simulink model "Robot2dof_control_Friction_FullyTuned_RBFNN"  (Simulink 8.5)
settings: Solver=ode45  StartTime=0.0  StopTime=20  RelTol=1e-3
values from neighbouring files (symbols this model uses):
  l1 = 1    [Inv_Kinematic.m]    (also in Parameters.m)
  l2 = 0.5    [Inv_Kinematic.m]    (also in Parameters.m)
  m1 = 2    [Parameters.m]
  m2 = 1    [Parameters.m]
libraries: mblibv1 x13
(part 1 of 2)
settings Model: Creator=Le Tien Dung  LastModifiedBy=Administrator
settings DebuggingCC: FcnCallInpInsideContextMsg=UseLocalSettings
settings SimMechanicsCC: VisOnUpdateDiagram=on  VisDuringSimulation=on
settings ConfigurationSet: Description=SimMechanics 2G

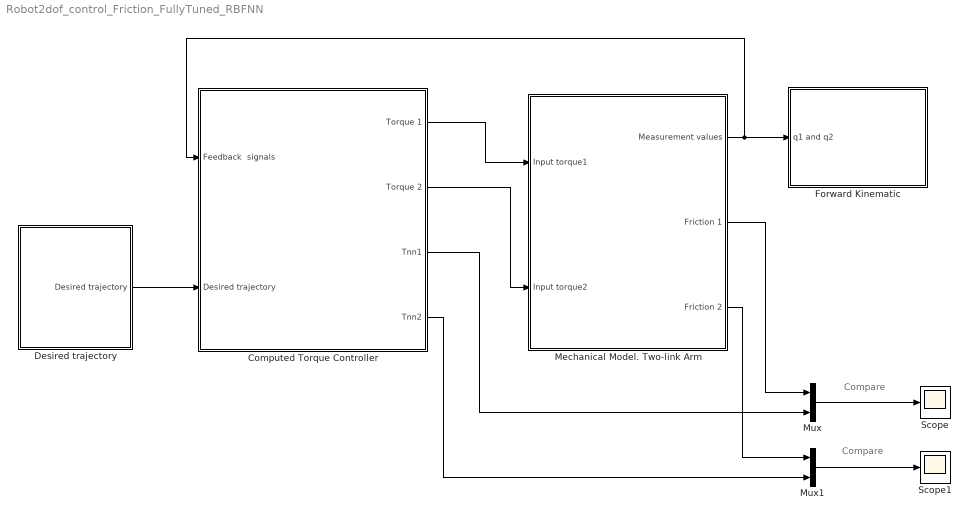
== system Robot2dof_control_Friction_FullyTuned_RBFNN ==
  note: Compare
  note: Compare
  Computed Torque Controller : Subsystem
  Desired trajectory : Subsystem
  Forward Kinematic : Subsystem
  Mechanical Model. Two-link Arm : Subsystem
  Mux : Mux  Inputs=2
  Mux1 : Mux  Inputs=2
  Scope : Scope
  Scope1 : Scope
      settings: SaveName=ScopeData2
  wires:
  Desired trajectory/1(Desired trajectory) -> Computed Torque Controller/2(Desired trajectory)
  Computed Torque Controller/1(Torque 1) -> Mechanical Model. Two-link Arm/1(Input torque1)
  Computed Torque Controller/2(Torque 2) -> Mechanical Model. Two-link Arm/2(Input torque2)
  Mux/1 -> Scope/1
  Mechanical Model. Two-link Arm/2(Friction 1) -> Mux/1
  Mux1/1 -> Scope1/1
  Mechanical Model. Two-link Arm/3(Friction 2) -> Mux1/1
  Mechanical Model. Two-link Arm/1(Measurement values) -> Computed Torque Controller/1(Feedback  signals), Forward Kinematic/1(q1 and q2)
  Computed Torque Controller/4(Tnn2) -> Mux1/2
  Computed Torque Controller/3(Tnn1) -> Mux/2

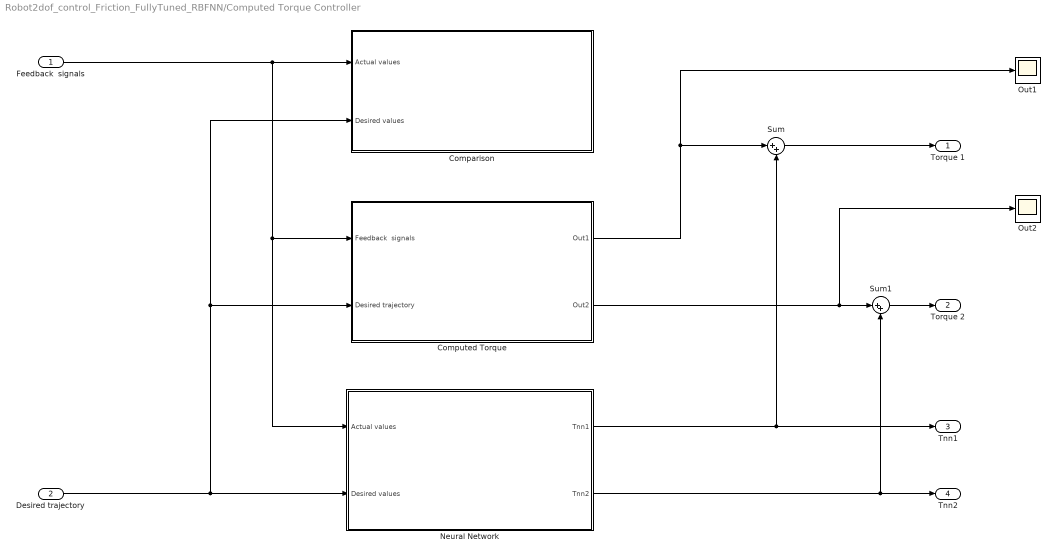
== system Robot2dof_control_Friction_FullyTuned_RBFNN/Computed Torque Controller ==
  Feedback  signals : Inport
  Desired trajectory : Inport  Port=2
  Comparison : Subsystem
  Computed Torque : Subsystem
  "Neural Network " : Subsystem
  Out1 : Scope
      settings: YMin=145.475  YMax=145.875  SaveName=Torque1
  Out2 : Scope
      settings: SaveName=Torque2
  Sum : Sum  Inputs=|++
  Sum1 : Sum  Inputs=|++
  Torque 1 : Outport
  Torque 2 : Outport  Port=2
  Tnn1 : Outport  Port=3
  Tnn2 : Outport  Port=4
  wires:
  Sum/1 -> Torque 1/1
  Sum1/1 -> Torque 2/1
  Computed Torque/1(Out1) -> Out1/1, Sum/1
  Computed Torque/2(Out2) -> Out2/1, Sum1/1
  Feedback  signals/1 -> Computed Torque/1(Feedback  signals), "Neural Network "/1("Actual values "), Comparison/1("Actual values ")
  Desired trajectory/1 -> "Neural Network "/2(Desired values), Comparison/2(Desired values), Computed Torque/2(Desired trajectory)
  "Neural Network "/1(Tnn1) -> Tnn1/1, Sum/2
  "Neural Network "/2(Tnn2) -> Tnn2/1, Sum1/2

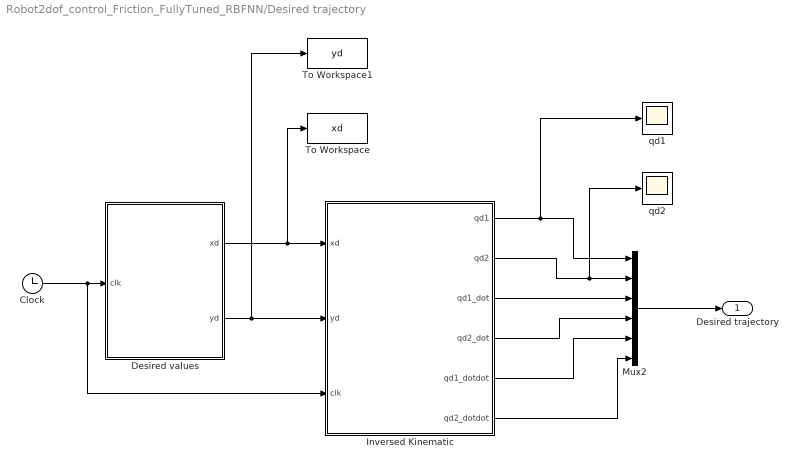
== system Robot2dof_control_Friction_FullyTuned_RBFNN/Desired trajectory ==
  " To Workspace1" : ToWorkspace  VariableName=yd  SaveFormat=Timeseries  SampleTime=-1
  Clock : Clock
  Desired values : MATLAB Function  TreatAsAtomicUnit=on
  Inversed Kinematic : MATLAB Function  TreatAsAtomicUnit=on
  Mux2 : Mux  Inputs=6
  To Workspace : ToWorkspace  VariableName=xd  SaveFormat=Timeseries  SampleTime=-1
  qd1 : Scope
  qd2 : Scope
      settings: SaveName=ScopeData3
  Desired trajectory : Outport
  wires:
  Mux2/1 -> Desired trajectory/1
  Desired values/1(xd) -> Inversed Kinematic/1(xd), To Workspace/1
  Clock/1 -> Desired values/1(clk), Inversed Kinematic/3(clk)
  Desired values/2(yd) -> Inversed Kinematic/2(yd), " To Workspace1"/1
  Inversed Kinematic/1(qd1) -> qd1/1, Mux2/1
  Inversed Kinematic/2(qd2) -> qd2/1, Mux2/2
  Inversed Kinematic/3(qd1_dot) -> Mux2/3
  Inversed Kinematic/4(qd2_dot) -> Mux2/4
  Inversed Kinematic/5(qd1_dotdot) -> Mux2/5
  Inversed Kinematic/6(qd2_dotdot) -> Mux2/6

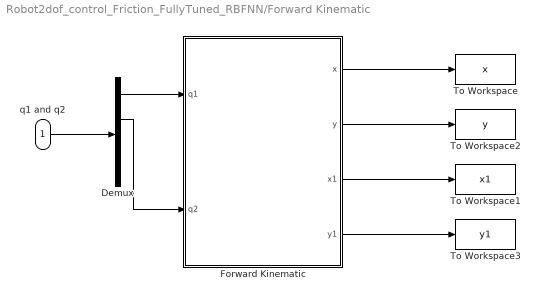
== system Robot2dof_control_Friction_FullyTuned_RBFNN/Forward Kinematic ==
  q1 and q2 : Inport
  Demux : Demux
  Forward Kinematic : MATLAB Function  TreatAsAtomicUnit=on
  To Workspace : ToWorkspace  VariableName=x  SaveFormat=Timeseries  SampleTime=-1
  To Workspace1 : ToWorkspace  VariableName=x1  SaveFormat=Timeseries  SampleTime=-1
  To Workspace2 : ToWorkspace  VariableName=y  SaveFormat=Timeseries  SampleTime=-1
  To Workspace3 : ToWorkspace  VariableName=y1  SaveFormat=Timeseries  SampleTime=-1
  wires:
  Forward Kinematic/4(y1) -> To Workspace3/1
  Demux/1 -> Forward Kinematic/1(q1)
  Forward Kinematic/2(y) -> To Workspace2/1
  Forward Kinematic/3(x1) -> To Workspace1/1
  Forward Kinematic/1(x) -> To Workspace/1
  Demux/2 -> Forward Kinematic/2(q2)
  q1 and q2/1 -> Demux/1

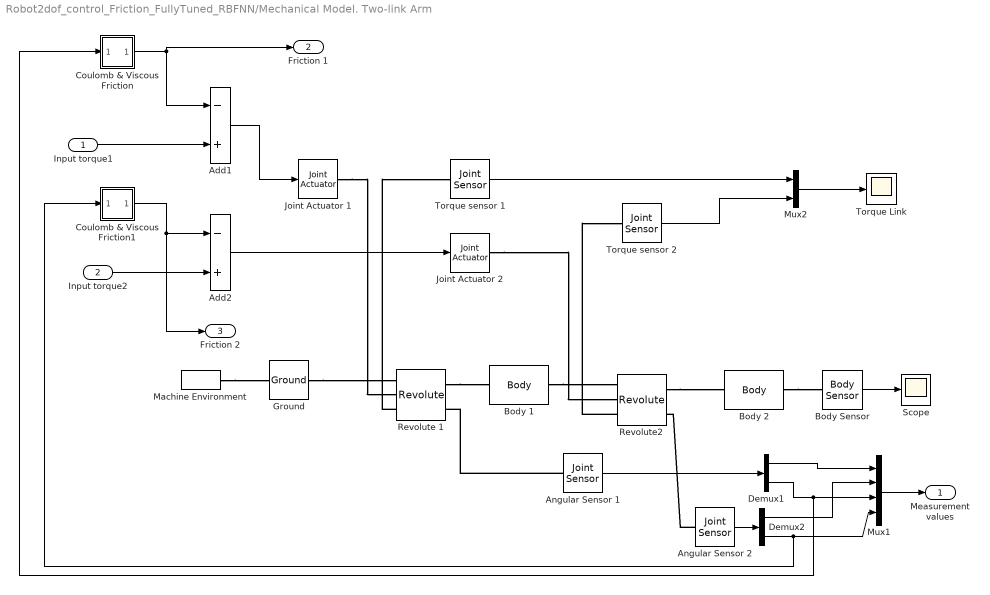
== system Robot2dof_control_Friction_FullyTuned_RBFNN/Mechanical Model. Two-link Arm ==
  Input torque1 : Inport
  Input torque2 : Inport  Port=2
  Add1 : Sum  Inputs=-+
  Add2 : Sum  Inputs=-+
  Angular Sensor 1 : mblibv1/Sensors &  Actuators/Joint Sensor  UpdateFromCAD=off  PhysicalDomain=Mechanical  PortType=blob  Muxed=on  Pose=off  Angle=on  AngleUnits=rad  ArcVelocity=on  ArcVelocityUnits=rad/s  ArcAcceleration=off  ArcAccelerationUnits=deg/s^2  CoordPosition=on  CoordPositionUnits=m  Velocity=off  VelocityUnits=m/s  Acceleration=off  AccelerationUnits=m/s^2  Quaternion=on  QuaternionDT=off  QuaternionDDT=off  QuaternionUnits=off  OutputVector=[1]  ActiveIO=on  Width=2  DialogClass=MechanicalSensorBlock  Primitive=R1  Force=off  ForceUnits=N  Torque=off  TorqueUnits=N*m  ReferenceFrame=Absolute (World)  ReactionSensedSide=Base  ReactionReferenceFrame=Absolute (World)  ReactionForce=off  ReactionForceUnits=N  ReactionMoment=off  ReactionMomentUnits=N*m
  Angular Sensor 2 : mblibv1/Sensors &  Actuators/Joint Sensor  UpdateFromCAD=off  PhysicalDomain=Mechanical  PortType=blob  Muxed=on  Pose=off  Angle=on  AngleUnits=rad  ArcVelocity=on  ArcVelocityUnits=rad/s  ArcAcceleration=off  ArcAccelerationUnits=deg/s^2  CoordPosition=on  CoordPositionUnits=m  Velocity=off  VelocityUnits=m/s  Acceleration=off  AccelerationUnits=m/s^2  Quaternion=on  QuaternionDT=off  QuaternionDDT=off  QuaternionUnits=off  OutputVector=[1]  ActiveIO=on  Width=2  DialogClass=MechanicalSensorBlock  Primitive=R1  Force=off  ForceUnits=N  Torque=off  TorqueUnits=N*m  ReferenceFrame=Absolute (World)  ReactionSensedSide=Base  ReactionReferenceFrame=Absolute (World)  ReactionForce=off  ReactionForceUnits=N  ReactionMoment=off  ReactionMomentUnits=N*m
  Body 1 : mblibv1/Bodies/Body  LConnTagsString=CS1  RConnTagsString=CS2  UpdateFromCAD=off  DialogClass=MechanicalBodyBlock  Mass=m1  MassUnits=kg  InertiaUnits=kg*m^2  Inertia=zeros(3,3)  Shape=Cylinder  ShapeDims=[1 1]  ShapeUnits=m  ShapeUse=false  Density=1  DensityUnits=kg/m^3  DensityUse=false  GraphicsMode=MACHINE_DEFAULT  BodyColorSelMode=MACHINE_DEFAULT  BodyColor=[1 0 0]  AttachedToCS=CG  CG=Left$CG$[l1/2 0 0]$World$World$m$[0 0 0]$Euler X-Y-Z$rad$World$false$none  WorkingFrames=Left$CS1$[0 0 0]$World$World$m$[0 0 0]$Euler X-Y-Z$rad$World$true$none#Right$CS2$[l1 0 0]$World$World$m$[0 0 0]$Euler X-Y-Z$rad$World$true$none  CGPos=[l1/2 0 0]  CGRot=[0 0 0]  CS0Pos=[]  CS0Rot=[]  CS1Pos=[0 0 0]  CS1Rot=[0 0 0]  CS2Pos=[l1 0 0]  CS2Rot=[0 0 0]  CS3Pos=[]  CS3Rot=[]  CS4Pos=[]  CS4Rot=[]  CS5Pos=[]  CS5Rot=[]  CS6Pos=[]  CS6Rot=[]  CS7Pos=[]  CS7Rot=[]  CS8Pos=[]  CS8Rot=[]  CS9Pos=[]  CS9Rot=[]  CS10Pos=[]  CS10Rot=[]  CS11Pos=[]  CS11Rot=[]  CS12Pos=[]  CS12Rot=[]  CS13Pos=[]  CS13Rot=[]  CS14Pos=[]  CS14Rot=[]  CS15Pos=[]  CS15Rot=[]  CS16Pos=[]  CS16Rot=[]  CS17Pos=[]  CS17Rot=[]  CS18Pos=[]  CS18Rot=[]  CS19Pos=[]  CS19Rot=[]  CS20Pos=[]  CS20Rot=[]
  Body 2 : mblibv1/Bodies/Body  LConnTagsString=CS1  RConnTagsString=CS2  UpdateFromCAD=off  DialogClass=MechanicalBodyBlock  Mass=m2  MassUnits=kg  InertiaUnits=kg*m^2  Inertia=zeros(3,3)  Shape=Cylinder  ShapeDims=[1 1]  ShapeUnits=m  ShapeUse=false  Density=1  DensityUnits=kg/m^3  DensityUse=false  GraphicsMode=MACHINE_DEFAULT  BodyColorSelMode=MACHINE_DEFAULT  BodyColor=[1 0 0]  AttachedToCS=CG  CG=Left$CG$[l2/2 0 0]$CS1$CS1$m$[0 0 0]$Euler X-Y-Z$rad$CS1$false$none  WorkingFrames=Left$CS1$[0 0 0]$Adjoining$Adjoining$m$[0 0 0]$Euler X-Y-Z$rad$Adjoining$true$none#Right$CS2$[l2 0 0]$CS1$CS1$m$[0 0 0]$Euler X-Y-Z$rad$CG$true$none  CGPos=[l2/2 0 0]  CGRot=[0 0 0]  CS0Pos=[]  CS0Rot=[]  CS1Pos=[0 0 0]  CS1Rot=[0 0 0]  CS2Pos=[l2 0 0]  CS2Rot=[0 0 0]  CS3Pos=[]  CS3Rot=[]  CS4Pos=[]  CS4Rot=[]  CS5Pos=[]  CS5Rot=[]  CS6Pos=[]  CS6Rot=[]  CS7Pos=[]  CS7Rot=[]  CS8Pos=[]  CS8Rot=[]  CS9Pos=[]  CS9Rot=[]  CS10Pos=[]  CS10Rot=[]  CS11Pos=[]  CS11Rot=[]  CS12Pos=[]  CS12Rot=[]  CS13Pos=[]  CS13Rot=[]  CS14Pos=[]  CS14Rot=[]  CS15Pos=[]  CS15Rot=[]  CS16Pos=[]  CS16Rot=[]  CS17Pos=[]  CS17Rot=[]  CS18Pos=[]  CS18Rot=[]  CS19Pos=[]  CS19Rot=[]  CS20Pos=[]  CS20Rot=[]
  Body Sensor : mblibv1/Sensors &  Actuators/Body Sensor  UpdateFromCAD=off  PhysicalDomain=Mechanical  PortType=blob  Muxed=on  Pose=off  Angle=on  AngleUnits=deg  ArcVelocity=off  ArcVelocityUnits=deg/s  ArcAcceleration=off  ArcAccelerationUnits=deg/s^2  CoordPosition=on  CoordPositionUnits=m  Velocity=off  VelocityUnits=m/s  Acceleration=off  AccelerationUnits=m/s^2  Quaternion=on  QuaternionDT=off  QuaternionDDT=off  QuaternionUnits=off  OutputVector=[1]  ActiveIO=on  Width=3  DialogClass=MechanicalSensorBlock  ReferenceFrame=Absolute (World)
  Coulomb & Viscous Friction : Subsystem  AncestorBlock=simulink/Discontinuities/Coulomb & Viscous Friction  mask(Coulombic and Viscous Friction){offset=0.3, gain=2}
      mask prompts: offset "Coulomb friction value (Offset):"; gain "Coefficient of viscous friction (Gain):"
      mask help:
      | A discontinuity offset at zero models coulomb friction.  Linear gain models viscous friction.
      | y = sign(x) * (Gain * abs(x) + Offset)
      mask init:
      | dblOffset = double(offset(1));
      | dblGain = double(gain(1));
      | x=max(dblOffset,dblGain+dblOffset);
      mask Help:
      | This block has a discontinuity
      | at zero and a linear gain afterward.
      | y= sign(x)*(Gain*abs(x)+Offset)
      mask Display:
      | plot([-1 0 0 1],[-dblGain-dblOffset, -dblOffset, ...
      |     dblOffset, dblGain+dblOffset],...
      |     [-1 1],[0 0],[0 0],[-x,x])
  Coulomb & Viscous Friction1 : Subsystem  AncestorBlock=simulink/Discontinuities/Coulomb & Viscous Friction  mask(Coulombic and Viscous Friction){offset=0.3, gain=2}
      mask prompts: offset "Coulomb friction value (Offset):"; gain "Coefficient of viscous friction (Gain):"
      mask help:
      | A discontinuity offset at zero models coulomb friction.  Linear gain models viscous friction.
      | y = sign(x) * (Gain * abs(x) + Offset)
      mask init:
      | dblOffset = double(offset(1));
      | dblGain = double(gain(1));
      | x=max(dblOffset,dblGain+dblOffset);
      mask Help:
      | This block has a discontinuity
      | at zero and a linear gain afterward.
      | y= sign(x)*(Gain*abs(x)+Offset)
      mask Display:
      | plot([-1 0 0 1],[-dblGain-dblOffset, -dblOffset, ...
      |     dblOffset, dblGain+dblOffset],...
      |     [-1 1],[0 0],[0 0],[-x,x])
  Demux1 : Demux  Outputs=2
  Demux2 : Demux  Outputs=2
  Ground : mblibv1/Bodies/Ground  UpdateFromCAD=off  LeftPortType=env  RightPortType=workingframe  PhysicalDomain=Mechanical  DialogClass=GroundBlock  CoordPosition=[0 0 0]  CoordPositionUnits=m  StateVectorMgrId=1  MachineId=[2 0]  ShowEnvPort=on  ParameterChecksum=[3725278248, 2799600244, 2519587858, 4125248297]  TopologyChecksum=[537926085, 4288578989, 2306256578, 2519465812]
  Joint Actuator 1 : mblibv1/Sensors &  Actuators/Joint Actuator  UpdateFromCAD=off  PhysicalDomain=Mechanical  PortType=blob  ActuationStyle=Force  AngleUnits=deg  ArcVelocityUnits=deg/s  ArcAccelerationUnits=deg/s^2  CoordPositionUnits=m  VelocityUnits=m/s  AccelerationUnits=m/s^2  ForceUnits=N  TorqueUnits=N*m  ActiveIO=on  Width=1  DialogClass=MechanicalActuatorBlock  Primitive=R1  ReferenceFrame=Absolute (World)
  Joint Actuator 2 : mblibv1/Sensors &  Actuators/Joint Actuator  UpdateFromCAD=off  PhysicalDomain=Mechanical  PortType=blob  ActuationStyle=Force  AngleUnits=deg  ArcVelocityUnits=deg/s  ArcAccelerationUnits=deg/s^2  CoordPositionUnits=m  VelocityUnits=m/s  AccelerationUnits=m/s^2  ForceUnits=N  TorqueUnits=N*m  ActiveIO=on  Width=1  DialogClass=MechanicalActuatorBlock  Primitive=R1  ReferenceFrame=Absolute (World)
  Machine Environment : mblibv1/Bodies/Machine Environment  PortType=env  PhysicalDomain=Mechanical  DialogTemplateClass=MECH.MachineEnvironment  SyncWhenCopied=off  Gravity=[0 -9.81 0]  GravityUnits=m/s^2  GravityAsSignal=off  Dimensionality=3D Only  AnalysisType=Forward dynamics  LinearAssemblyTolerance=1e-3  LinearAssemblyToleranceUnits=m  AngularAssemblyTolerance=1e-3  AngularAssemblyToleranceUnits=rad  ConstraintSolverType=Stabilizing  ConstraintRelTolerance=1e-4  ConstraintAbsTolerance=1e-4  UseRobustSingularityHandling=off  RedundancyAnalysisToleranceType=Automatically select tolerance  RedundancyAnalysisTolerance=1e-14  StatePerturbationType=Fixed  PerturbationSize=1e-5  VisualizeMachine=on  BodyVisualizationType=Use model default body geometries  BodyColorSelMode=Use model default  DefaultBodyColor=[1 0 0]
  Mux1 : Mux
  Mux2 : Mux  Inputs=2
  Revolute 1 : mblibv1/Joints/Revolute  LConnTagsString=__newl0|SA1|SA2  RConnTagsString=__newr0|SA1  UpdateFromCAD=off  NumSAPorts=3  CutJoint=off  MarkAsCut=off  Primitives=prismatic  PrimitiveProps=R1$World$[0 0 1]$revolute  DialogClass=JointBlock  R1Axis=[0 0 1]
  Revolute2 : mblibv1/Joints/Revolute  LConnTagsString=__newl0|SA1|SA2  RConnTagsString=__newr0|SA1  UpdateFromCAD=off  NumSAPorts=3  CutJoint=off  MarkAsCut=off  Primitives=prismatic  PrimitiveProps=R1$Base$[0 0 1]$revolute  DialogClass=JointBlock  R1Axis=[0 0 1]
  Scope : Scope
      settings: SaveName=ScopeData6
  Torque Link : Scope
      settings: SaveName=Torq1_task
  Torque sensor 1 : mblibv1/Sensors &  Actuators/Joint Sensor  UpdateFromCAD=off  PhysicalDomain=Mechanical  PortType=blob  Muxed=on  Pose=off  Angle=off  AngleUnits=rad  ArcVelocity=off  ArcVelocityUnits=rad/s  ArcAcceleration=off  ArcAccelerationUnits=deg/s^2  CoordPosition=on  CoordPositionUnits=m  Velocity=off  VelocityUnits=m/s  Acceleration=off  AccelerationUnits=m/s^2  Quaternion=on  QuaternionDT=off  QuaternionDDT=off  QuaternionUnits=off  OutputVector=[1]  ActiveIO=on  Width=1  DialogClass=MechanicalSensorBlock  Primitive=R1  Force=off  ForceUnits=N  Torque=on  TorqueUnits=N*m  ReferenceFrame=Absolute (World)  ReactionSensedSide=Base  ReactionReferenceFrame=Absolute (World)  ReactionForce=off  ReactionForceUnits=N  ReactionMoment=off  ReactionMomentUnits=N*m
  Torque sensor 2 : mblibv1/Sensors &  Actuators/Joint Sensor  UpdateFromCAD=off  PhysicalDomain=Mechanical  PortType=blob  Muxed=on  Pose=off  Angle=off  AngleUnits=rad  ArcVelocity=off  ArcVelocityUnits=rad/s  ArcAcceleration=off  ArcAccelerationUnits=deg/s^2  CoordPosition=on  CoordPositionUnits=m  Velocity=off  VelocityUnits=m/s  Acceleration=off  AccelerationUnits=m/s^2  Quaternion=on  QuaternionDT=off  QuaternionDDT=off  QuaternionUnits=off  OutputVector=[1]  ActiveIO=on  Width=1  DialogClass=MechanicalSensorBlock  Primitive=R1  Force=off  ForceUnits=N  Torque=on  TorqueUnits=N*m  ReferenceFrame=Absolute (World)  ReactionSensedSide=Base  ReactionReferenceFrame=Absolute (World)  ReactionForce=off  ReactionForceUnits=N  ReactionMoment=off  ReactionMomentUnits=N*m
  Measurement values : Outport
  Friction 1 : Outport  Port=2
  Friction 2 : Outport  Port=3
  wires:
  Angular Sensor 1/1 -> Demux1/1
  Angular Sensor 2/1 -> Demux2/1
  Mux2/1 -> Torque Link/1
  Torque sensor 2/1 -> Mux2/2
  Torque sensor 1/1 -> Mux2/1
  Demux1/1 -> Mux1/1
  Demux2/1 -> Mux1/2
  Demux1/2 -> Mux1/3, Coulomb & Viscous Friction/1(In1)
  Demux2/2 -> Mux1/4, Coulomb & Viscous Friction1/1(In1)
  Mux1/1 -> Measurement values/1
  Add1/1 -> Joint Actuator 1/1
  Coulomb & Viscous Friction/1(Out1) -> Add1/1, Friction 1/1
  Input torque1/1 -> Add1/2
  Input torque2/1 -> Add2/2
  Add2/1 -> Joint Actuator 2/1
  Coulomb & Viscous Friction1/1(Out1) -> Add2/1, Friction 2/1
  Body Sensor/1 -> Scope/1
  connections:
  Revolute 1/RConn1 -- Body 1/LConn1
  Body 1/RConn1 -- Revolute2/LConn1
  Machine Environment/RConn1 -- Ground/LConn1
  Ground/RConn1 -- Revolute 1/LConn1
  Joint Actuator 1/RConn1 -- Revolute 1/LConn2
  Joint Actuator 2/RConn1 -- Revolute2/LConn2
  Angular Sensor 1/LConn1 -- Revolute 1/RConn2
  Angular Sensor 2/LConn1 -- Revolute2/RConn2
  Revolute2/LConn3 -- Torque sensor 2/LConn1
  Revolute 1/LConn3 -- Torque sensor 1/LConn1
  Body 2/RConn1 -- Body Sensor/LConn1
  Revolute2/RConn1 -- Body 2/LConn1

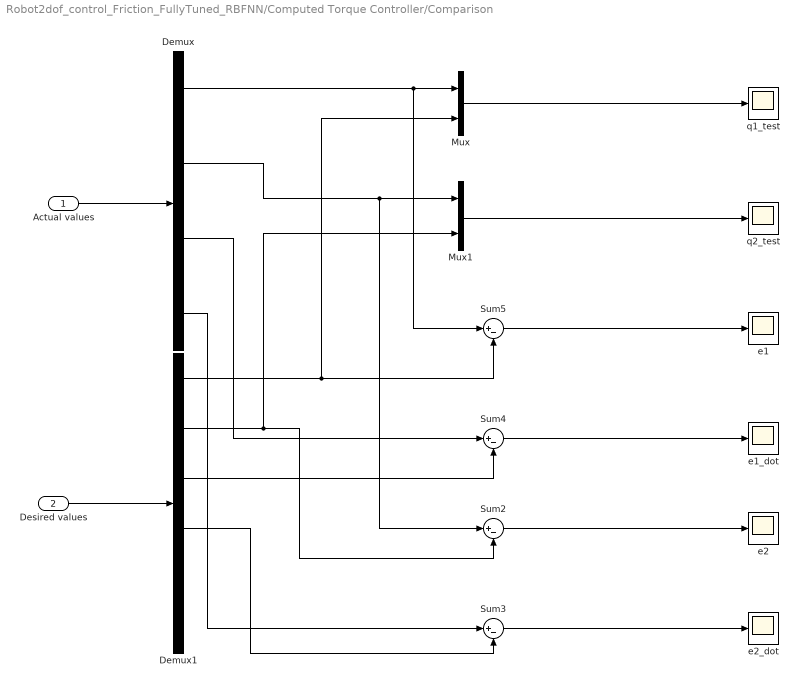
== system Robot2dof_control_Friction_FullyTuned_RBFNN/Computed Torque Controller/Comparison ==
  "Actual values " : Inport
  Desired values : Inport  Port=2
  Demux : Demux
  Demux1 : Demux  Outputs=6
  Mux : Mux  Inputs=2
  Mux1 : Mux  Inputs=2
  Sum{2..5} (4 alike) : Sum  Inputs=|+-
  e1 : Scope
      settings: ShowLegends=on  TimeRange=20  YMin=-1.4  YMax=0.3999999999999999  SaveName=Joint3
  e1_dot : Scope
      settings: TimeRange=20  YMin=-1  YMax=3  SaveName=Joint
  e2 : Scope
      settings: ShowLegends=on  TimeRange=19.57401979042055  YMin=-1.5  YMax=2.5  SaveName=Joint4
  e2_dot : Scope
      settings: YMax=3  SaveName=Joint5
  q1_test : Scope
      settings: ShowLegends=on  TimeRange=20  YMin=-0.002137407065588336  YMax=2  SaveName=Joint6
  q2_test : Scope
      settings: ShowLegends=on  TimeRange=20  YMin=-3.25  YMax=1.5  SaveName=Joint7
  wires:
  Mux1/1 -> q2_test/1
  Sum3/1 -> e2_dot/1
  Sum5/1 -> e1/1
  Sum4/1 -> e1_dot/1
  Sum2/1 -> e2/1
  Desired values/1 -> Demux1/1
  "Actual values "/1 -> Demux/1
  Mux/1 -> q1_test/1
  Demux/1 -> Sum5/1, Mux/1
  Demux1/1 -> Sum5/2, Mux/2
  Demux/2 -> Sum2/1, Mux1/1
  Demux1/2 -> Sum2/2, Mux1/2
  Demux/3 -> Sum4/1
  Demux1/3 -> Sum4/2
  Demux/4 -> Sum3/1
  Demux1/4 -> Sum3/2

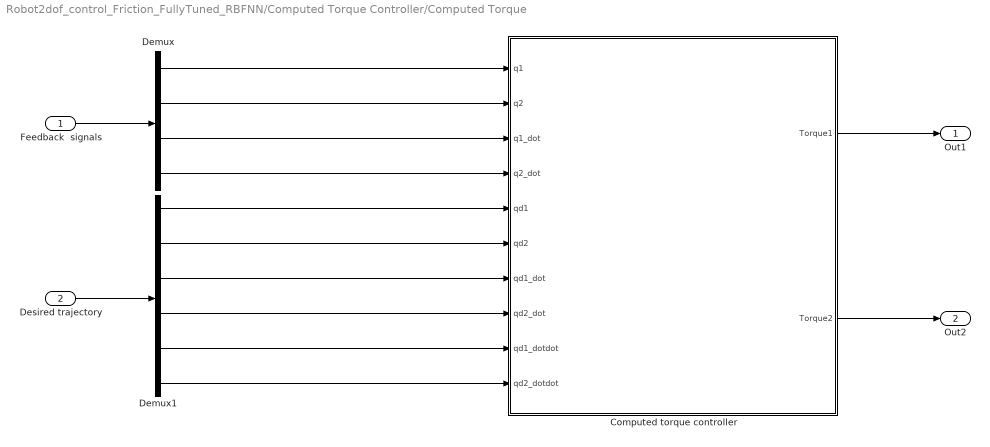
== system Robot2dof_control_Friction_FullyTuned_RBFNN/Computed Torque Controller/Computed Torque ==
  Feedback  signals : Inport
  Desired trajectory : Inport  Port=2
  Computed torque controller : MATLAB Function  TreatAsAtomicUnit=on
  Demux : Demux
  Demux1 : Demux  Outputs=6
  Out1 : Outport
  Out2 : Outport  Port=2
  wires:
  Computed torque controller/2(Torque2) -> Out2/1
  Computed torque controller/1(Torque1) -> Out1/1
  Demux/1 -> Computed torque controller/1(q1)
  Demux/2 -> Computed torque controller/2(q2)
  Demux/3 -> Computed torque controller/3(q1_dot)
  Demux/4 -> Computed torque controller/4(q2_dot)
  Demux1/1 -> Computed torque controller/5(qd1)
  Demux1/2 -> Computed torque controller/6(qd2)
  Demux1/3 -> Computed torque controller/7(qd1_dot)
  Demux1/4 -> Computed torque controller/8(qd2_dot)
  Demux1/5 -> Computed torque controller/9(qd1_dotdot)
  Demux1/6 -> Computed torque controller/10(qd2_dotdot)
  Feedback  signals/1 -> Demux/1
  Desired trajectory/1 -> Demux1/1

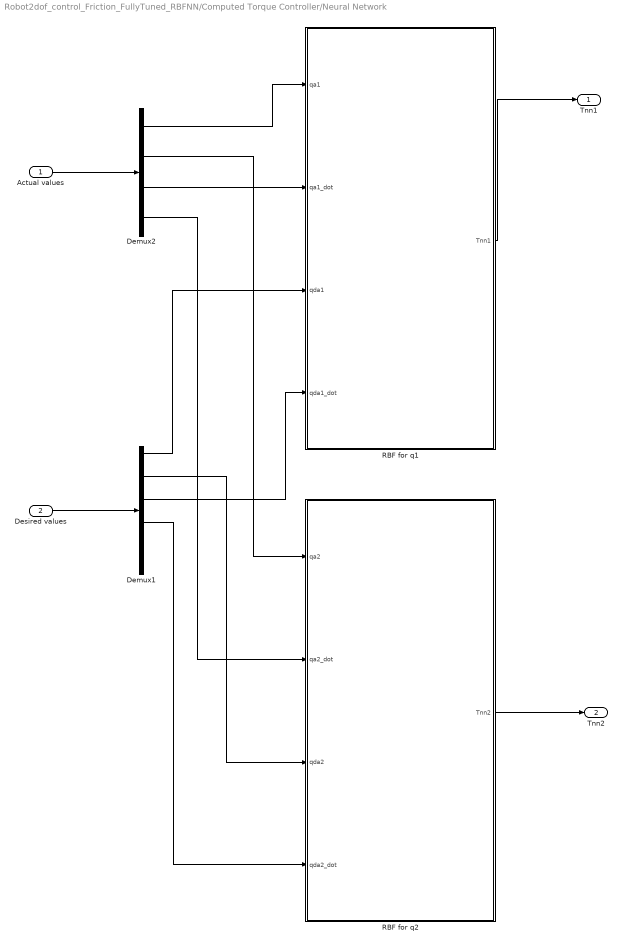
== system Robot2dof_control_Friction_FullyTuned_RBFNN/Computed Torque Controller/Neural Network  ==
  "Actual values " : Inport
  Desired values : Inport  Port=2
  Demux1 : Demux  Outputs=6
  Demux2 : Demux
  RBF for q1 : MATLAB Function  TreatAsAtomicUnit=on
  RBF for q2 : MATLAB Function  TreatAsAtomicUnit=on
  Tnn1 : Outport
  Tnn2 : Outport  Port=2
  wires:
  RBF for q1/1(Tnn1) -> Tnn1/1
  "Actual values "/1 -> Demux2/1
  RBF for q2/1(Tnn2) -> Tnn2/1
  Demux2/2 -> RBF for q2/1(qa2)
  Demux2/4 -> RBF for q2/2(qa2_dot)
  Demux2/1 -> RBF for q1/1(qa1)
  Demux2/3 -> RBF for q1/2(qa1_dot)
  Desired values/1 -> Demux1/1
  Demux1/1 -> RBF for q1/3(qda1)
  Demux1/4 -> RBF for q2/4(qda2_dot)
  Demux1/2 -> RBF for q2/3(qda2)
  Demux1/3 -> RBF for q1/4(qda1_dot)

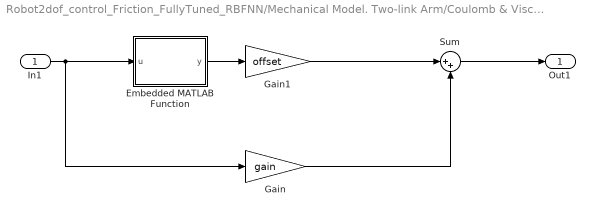
== system Robot2dof_control_Friction_FullyTuned_RBFNN/Mechanical Model. Two-link Arm/Coulomb & Viscous Friction ==
  In1 : Inport
  Embedded MATLAB Function : MATLAB Function  TreatAsAtomicUnit=on
  Gain : Gain  DisableCoverage=on  Gain=gain  SaturateOnIntegerOverflow=on  OutDataTypeStr=Inherit: Same as input
  Gain1 : Gain  DisableCoverage=on  Gain=offset  OutDataTypeStr=Inherit: Inherit via back propagation  SaturateOnIntegerOverflow=on
  Sum : Sum  Inputs=|++  SaturateOnIntegerOverflow=on  InputSameDT=on  OutDataTypeStr=Inherit: Same as first input
  Out1 : Outport
  wires:
  Embedded MATLAB Function/1(y) -> Gain1/1
  In1/1 -> Embedded MATLAB Function/1(u), Gain/1
  Gain1/1 -> Sum/1
  Sum/1 -> Out1/1
  Gain/1 -> Sum/2

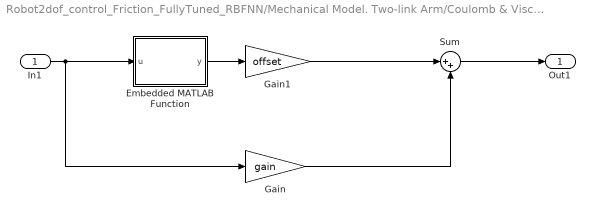
== system Robot2dof_control_Friction_FullyTuned_RBFNN/Mechanical Model. Two-link Arm/Coulomb & Viscous Friction1 ==
  In1 : Inport
  Embedded MATLAB Function : MATLAB Function  TreatAsAtomicUnit=on
  Gain : Gain  DisableCoverage=on  Gain=gain  SaturateOnIntegerOverflow=on  OutDataTypeStr=Inherit: Same as input
  Gain1 : Gain  DisableCoverage=on  Gain=offset  OutDataTypeStr=Inherit: Inherit via back propagation  SaturateOnIntegerOverflow=on
  Sum : Sum  Inputs=|++  SaturateOnIntegerOverflow=on  InputSameDT=on  OutDataTypeStr=Inherit: Same as first input
  Out1 : Outport
  wires:
  Gain/1 -> Sum/2
  Sum/1 -> Out1/1
  Gain1/1 -> Sum/1
  In1/1 -> Gain/1, Embedded MATLAB Function/1(u)
  Embedded MATLAB Function/1(y) -> Gain1/1

== matlab function Mechanical Model. Two-link Arm/Coulomb & Viscous Friction1/Embedded MATLAB Function ==
  data: u input double; y output double
function y = Sat(u)

if (abs(u)>0.01)
    y = sign(u);
else
    y = u/0.01;
end

== matlab function Desired trajectory/Desired values ==
  data: xd output double; yd output double; clk input double
function [xd, yd] = Desired_values(clk)
%% Parameters
T=5;
x0 = sqrt(2)/2;
y0 = sqrt(2)/2;
R = 0.5;
w = 2*pi/T;

%% Desired values
    xd = x0 + R*cos(w*clk +pi/2);
    yd = y0 + R*sin(w*clk +pi/2);
    
end

== matlab function Forward Kinematic/Forward Kinematic ==
  data: q1 input double; q2 input double; x output double; y output double; x1 output double; y1 output double
function [x,y,x1,y1]= Forward_Kinematic(q1, q2)
%% Parameters    
l1=1; 
l2=0.5;

%% Compute
x = l1*cos(q1) +l2*cos(q1+q2);
y = l1*sin(q1) +l2*sin(q1+q2);
x1 = l1*cos(q1);
y1 = l1*sin(q1);

== matlab function Desired trajectory/Inversed Kinematic ==
  data: xd input double; yd input double; qd1 output double; qd2 output double; qd1_dot output double; qd2_dot output double; clk input double; qd1_dotdot output double; qd2_dotdot output double
function [qd1, qd2, qd1_dot, qd2_dot, qd1_dotdot, qd2_dotdot] = InvKinematic( xd, yd, clk )
%% Parameters
x0 = sqrt(2)/2;
y0 = sqrt(2)/2;
l1 = 1;
l2 = 0.5;
T=5;
R = 0.5;
w = 2*pi/T;
x1 = 0;
y1= 0;
x = 0;
y= 0;
qd1 = 0;
qd2 = 0;


%% Inversed Kinematic
   qd2 = acos((xd^2 + yd^2 - l1^2 - l2^2)/(2*l1*l2));
   if(qd2 > 0)
       qd2 = -qd2;
       qd2_dot = ((2*pi*cos(pi/2 + (2*pi*clk)/5)*(sin(pi/2 + (2*pi*clk)/5)/2 + 2^(1/2)/2))/5 - (2*pi*sin(pi/2 + (2*pi*clk)/5)*(cos(pi/2 + (2*pi*clk)/5)/2 + 2^(1/2)/2))/5)/(- ((cos(pi/2 + (2*pi*clk)/5)/2 + 2^(1/2)/2)^2 + (sin(pi/2 + (2*pi*clk)/5)/2 + 2^(1/2)/2)^2 - 5/4)^2 + 1)^(1/2);
       qd2_dotdot = ((2*pi^2*sin(pi/2 + (2*pi*clk)/5)^2)/25 + (2*pi^2*cos(pi/2 + (2*pi*clk)/5)^2)/25 - (4*pi^2*cos(pi/2 + (2*pi*clk)/5)*(cos(pi/2 + (2*pi*clk)/5)/2 + 2^(1/2)/2))/25 - (4*pi^2*sin(pi/2 + (2*pi*clk)/5)*(sin(pi/2 + (2*pi*clk)/5)/2 + 2^(1/2)/2))/25)/(- ((cos(pi/2 + (2*pi*clk)/5)/2 + 2^(1/2)/2)^2 + (sin(pi/2 + (2*pi*clk)/5)/2 + 2^(1/2)/2)^2 - 5/4)^2 + 1)^(1/2) + (((2*pi*cos(pi/2 + (2*pi*clk)/5)*(sin(pi/2 + (2*pi*clk)/5)/2 + 2^(1/2)/2))/5 - (2*pi*sin(pi/2 + (2*pi*clk)/5)*(cos(pi/2 + (2*pi*clk)/5)/2 + 2^(1/2)/2))/5)^2*((cos(pi/2 + (2*pi*clk)/5)/2 + 2^(1/2)/2)^2 + (sin(pi/2 + (2*pi*clk)/5)/2 + 2^(1/2)/2)^2 - 5/4))/(- ((cos(pi/2 + (2*pi*clk)/5)/2 + 2^(1/2)/2)^2 + (sin(pi/2 + (2*pi*clk)/5)/2 + 2^(1/2)/2)^2 - 5/4)^2 + 1)^(3/2);
        
   else
       qd2=qd2;
        qd2_dot = -((2*pi*cos(pi/2 + (2*pi*clk)/5)*(sin(pi/2 + (2*pi*clk)/5)/2 + 2^(1/2)/2))/5 - (2*pi*sin(pi/2 + (2*pi*clk)/5)*(cos(pi/2 + (2*pi*clk)/5)/2 + 2^(1/2)/2))/5)/(- ((cos(pi/2 + (2*pi*clk)/5)/2 + 2^(1/2)/2)^2 + (sin(pi/2 + (2*pi*clk)/5)/2 + 2^(1/2)/2)^2 - 5/4)^2 + 1)^(1/2);
        qd2_dotdot = - ((2*pi^2*sin(pi/2 + (2*pi*clk)/5)^2)/25 + (2*pi^2*cos(pi/2 + (2*pi*clk)/5)^2)/25 - (4*pi^2*cos(pi/2 + (2*pi*clk)/5)*(cos(pi/2 + (2*pi*clk)/5)/2 + 2^(1/2)/2))/25 - (4*pi^2*sin(pi/2 + (2*pi*clk)/5)*(sin(pi/2 + (2*pi*clk)/5)/2 + 2^(1/2)/2))/25)/(- ((cos(pi/2 + (2*pi*clk)/5)/2 + 2^(1/2)/2)^2 + (sin(pi/2 + (2*pi*clk)/5)/2 + 2^(1/2)/2)^2 - 5/4)^2 + 1)^(1/2) - (((2*pi*cos(pi/2 + (2*pi*clk)/5)*(sin(pi/2 + (2*pi*clk)/5)/2 + 2^(1/2)/2))/5 - (2*pi*sin(pi/2 + (2*pi*clk)/5)*(cos(pi/2 + (2*pi*clk)/5)/2 + 2^(1/2)/2))/5)^2*((cos(pi/2 + (2*pi*clk)/5)/2 + 2^(1/2)/2)^2 + (sin(pi/2 + (2*pi*clk)/5)/2 + 2^(1/2)/2)^2 - 5/4))/(- ((cos(pi/2 + (2*pi*clk)/5)/2 + 2^(1/2)/2)^2 + (sin(pi/2 + (2*pi*clk)/5)/2 + 2^(1/2)/2)^2 - 5/4)^2 + 1)^(3/2);
        
   end
   
   qd1 = asin((yd*(l1+l2*cos(qd2))-xd*l2*sin(qd2))/(xd^2+yd^2));
      
       x = l1*cos(qd1) +l2*cos(qd1+qd2);
       if((x-xd)<0.01 || (x-xd)<-0.01)
        
            qd1 = qd1;
            qd1_dot = (((sin(pi/2 + (2*pi*clk)/5)/2 + 2^(1/2)/2)*((pi*cos(pi/2 + (2*pi*clk)/5)*(sin(pi/2 + (2*pi*clk)/5)/2 + 2^(1/2)/2))/5 - (pi*sin(pi/2 + (2*pi*clk)/5)*(cos(pi/2 + (2*pi*clk)/5)/2 + 2^(1/2)/2))/5) + (pi*cos(pi/2 + (2*pi*clk)/5)*((cos(pi/2 + (2*pi*clk)/5)/2 + 2^(1/2)/2)^2/2 + (sin(pi/2 + (2*pi*clk)/5)/2 + 2^(1/2)/2)^2/2 + 3/8))/5 + (pi*sin(pi/2 + (2*pi*clk)/5)*(1 - ((cos(pi/2 + (2*pi*clk)/5)/2 + 2^(1/2)/2)^2 + (sin(pi/2 + (2*pi*clk)/5)/2 + 2^(1/2)/2)^2 - 5/4)^2)^(1/2))/10 + ((cos(pi/2 + (2*pi*clk)/5)/4 + 2^(1/2)/4)*((2*pi*cos(pi/2 + (2*pi*clk)/5)*(sin(pi/2 + (2*pi*clk)/5)/2 + 2^(1/2)/2))/5 - (2*pi*sin(pi/2 + (2*pi*clk)/5)*(cos(pi/2 + (2*pi*clk)/5)/2 + 2^(1/2)/2))/5)*((cos(pi/2 + (2*pi*clk)/5)/2 + 2^(1/2)/2)^2 + (sin(pi/2 + (2*pi*clk)/5)/2 + 2^(1/2)/2)^2 - 5/4))/(1 - ((cos(pi/2 + (2*pi*clk)/5)/2 + 2^(1/2)/2)^2 + (sin(pi/2 + (2*pi*clk)/5)/2 + 2^(1/2)/2)^2 - 5/4)^2)^(1/2))/((cos(pi/2 + (2*pi*clk)/5)/2 + 2^(1/2)/2)^2 + (sin(pi/2 + (2*pi*clk)/5)/2 + 2^(1/2)/2)^2) + (((cos(pi/2 + (2*pi*clk)/5)/4 + 2^(1/2)/4)*(1 - ((cos(pi/2 + (2*pi*clk)/5)/2 + 2^(1/2)/2)^2 + (sin(pi/2 + (2*pi*clk)/5)/2 + 2^(1/2)/2)^2 - 5/4)^2)^(1/2) - (sin(pi/2 + (2*pi*clk)/5)/2 + 2^(1/2)/2)*((cos(pi/2 + (2*pi*clk)/5)/2 + 2^(1/2)/2)^2/2 + (sin(pi/2 + (2*pi*clk)/5)/2 + 2^(1/2)/2)^2/2 + 3/8))*((2*pi*cos(pi/2 + (2*pi*clk)/5)*(sin(pi/2 + (2*pi*clk)/5)/2 + 2^(1/2)/2))/5 - (2*pi*sin(pi/2 + (2*pi*clk)/5)*(cos(pi/2 + (2*pi*clk)/5)/2 + 2^(1/2)/2))/5))/((cos(pi/2 + (2*pi*clk)/5)/2 + 2^(1/2)/2)^2 + (sin(pi/2 + (2*pi*clk)/5)/2 + 2^(1/2)/2)^2)^2)/(1 - ((cos(pi/2 + (2*pi*clk)/5)/4 + 2^(1/2)/4)*(1 - ((cos(pi/2 + (2*pi*clk)/5)/2 + 2^(1/2)/2)^2 + (sin(pi/2 + (2*pi*clk)/5)/2 + 2^(1/2)/2)^2 - 5/4)^2)^(1/2) - (sin(pi/2 + (2*pi*clk)/5)/2 + 2^(1/2)/2)*((cos(pi/2 + (2*pi*clk)/5)/2 + 2^(1/2)/2)^2/2 + (sin(pi/2 + (2*pi*clk)/5)/2 + 2^(1/2)/2)^2/2 + 3/8))^2/((cos(pi/2 + (2*clk*pi)/5)/2 + 2^(1/2)/2)^2 + (sin(pi/2 + (2*clk*pi)/5)/2 + 2^(1/2)/2)^2)^2)^(1/2);
            qd1_dotdot = (((sin(pi/2 + (2*pi*clk)/5)/2 + 2^(1/2)/2)*((pi^2*sin(pi/2 + (2*pi*clk)/5)^2)/25 + (pi^2*cos(pi/2 + (2*pi*clk)/5)^2)/25 - (2*pi^2*cos(pi/2 + (2*pi*clk)/5)*(cos(pi/2 + (2*pi*clk)/5)/2 + 2^(1/2)/2))/25 - (2*pi^2*sin(pi/2 + (2*pi*clk)/5)*(sin(pi/2 + (2*pi*clk)/5)/2 + 2^(1/2)/2))/25) + (2*pi*cos(pi/2 + (2*pi*clk)/5)*((pi*cos(pi/2 + (2*pi*clk)/5)*(sin(pi/2 + (2*pi*clk)/5)/2 + 2^(1/2)/2))/5 - (pi*sin(pi/2 + (2*pi*clk)/5)*(cos(pi/2 + (2*pi*clk)/5)/2 + 2^(1/2)/2))/5))/5 + (pi^2*cos(pi/2 + (2*pi*clk)/5)*(1 - ((cos(pi/2 + (2*pi*clk)/5)/2 + 2^(1/2)/2)^2 + (sin(pi/2 + (2*pi*clk)/5)/2 + 2^(1/2)/2)^2 - 5/4)^2)^(1/2))/25 + ((cos(pi/2 + (2*pi*clk)/5)/4 + 2^(1/2)/4)*((2*pi*cos(pi/2 + (2*pi*clk)/5)*(sin(pi/2 + (2*pi*clk)/5)/2 + 2^(1/2)/2))/5 - (2*pi*sin(pi/2 + (2*pi*clk)/5)*(cos(pi/2 + (2*pi*clk)/5)/2 + 2^(1/2)/2))/5)^2)/(1 - ((cos(pi/2 + (2*pi*clk)/5)/2 + 2^(1/2)/2)^2 + (sin(pi/2 + (2*pi*clk)/5)/2 + 2^(1/2)/2)^2 - 5/4)^2)^(1/2) - (2*pi^2*sin(pi/2 + (2*pi*clk)/5)*((cos(pi/2 + (2*pi*clk)/5)/2 + 2^(1/2)/2)^2/2 + (sin(pi/2 + (2*pi*clk)/5)/2 + 2^(1/2)/2)^2/2 + 3/8))/25 + ((cos(pi/2 + (2*pi*clk)/5)/4 + 2^(1/2)/4)*((cos(pi/2 + (2*pi*clk)/5)/2 + 2^(1/2)/2)^2 + (sin(pi/2 + (2*pi*clk)/5)/2 + 2^(1/2)/2)^2 - 5/4)*((2*pi^2*sin(pi/2 + (2*pi*clk)/5)^2)/25 + (2*pi^2*cos(pi/2 + (2*pi*clk)/5)^2)/25 - (4*pi^2*cos(pi/2 + (2*pi*clk)/5)*(cos(pi/2 + (2*pi*clk)/5)/2 + 2^(1/2)/2))/25 - (4*pi^2*sin(pi/2 + (2*pi*clk)/5)*(sin(pi/2 + (2*pi*clk)/5)/2 + 2^(1/2)/2))/25))/(1 - ((cos(pi/2 + (2*pi*clk)/5)/2 + 2^(1/2)/2)^2 + (sin(pi/2 + (2*pi*clk)/5)/2 + 2^(1/2)/2)^2 - 5/4)^2)^(1/2) + ((cos(pi/2 + (2*pi*clk)/5)/4 + 2^(1/2)/4)*((2*pi*cos(pi/2 + (2*pi*clk)/5)*(sin(pi/2 + (2*pi*clk)/5)/2 + 2^(1/2)/2))/5 - (2*pi*sin(pi/2 + (2*pi*clk)/5)*(cos(pi/2 + (2*pi*clk)/5)/2 + 2^(1/2)/2))/5)^2*((cos(pi/2 + (2*pi*clk)/5)/2 + 2^(1/2)/2)^2 + (sin(pi/2 + (2*pi*clk)/5)/2 + 2^(1/2)/2)^2 - 5/4)^2)/(1 - ((cos(pi/2 + (2*pi*clk)/5)/2 + 2^(1/2)/2)^2 + (sin(pi/2 + (2*pi*clk)/5)/2 + 2^(1/2)/2)^2 - 5/4)^2)^(3/2) - (pi*sin(pi/2 + (2*pi*clk)/5)*((2*pi*cos(pi/2 + (2*pi*clk)/5)*(sin(pi/2 + (2*pi*clk)/5)/2 + 2^(1/2)/2))/5 - (2*pi*sin(pi/2 + (2*pi*clk)/5)*(cos(pi/2 + (2*pi*clk)/5)/2 + 2^(1/2)/2))/5)*((cos(pi/2 + (2*pi*clk)/5)/2 + 2^(1/2)/2)^2 + (sin(pi/2 + (2*pi*clk)/5)/2 + 2^(1/2)/2)^2 - 5/4))/(5*(1 - ((cos(pi/2 + (2*pi*clk)/5)/2 + 2^(1/2)/2)^2 + (sin(pi/2 + (2*pi*clk)/5)/2 + 2^(1/2)/2)^2 - 5/4)^2)^(1/2)))/((cos(pi/2 + (2*pi*clk)/5)/2 + 2^(1/2)/2)^2 + (sin(pi/2 + (2*pi*clk)/5)/2 + 2^(1/2)/2)^2) - (2*((2*pi*cos(pi/2 + (2*pi*clk)/5)*(sin(pi/2 + (2*pi*clk)/5)/2 + 2^(1/2)/2))/5 - (2*pi*sin(pi/2 + (2*pi*clk)/5)*(cos(pi/2 + (2*pi*clk)/5)/2 + 2^(1/2)/2))/5)*((sin(pi/2 + (2*pi*clk)/5)/2 + 2^(1/2)/2)*((pi*cos(pi/2 + (2*pi*clk)/5)*(sin(pi/2 + (2*pi*clk)/5)/2 + 2^(1/2)/2))/5 - (pi*sin(pi/2 + (2*pi*clk)/5)*(cos(pi/2 + (2*pi*clk)/5)/2 + 2^(1/2)/2))/5) + (pi*cos(pi/2 + (2*pi*clk)/5)*((cos(pi/2 + (2*pi*clk)/5)/2 + 2^(1/2)/2)^2/2 + (sin(pi/2 + (2*pi*clk)/5)/2 + 2^(1/2)/2)^2/2 + 3/8))/5 + (pi*sin(pi/2 + (2*pi*clk)/5)*(1 - ((cos(pi/2 + (2*pi*clk)/5)/2 + 2^(1/2)/2)^2 + (sin(pi/2 + (2*pi*clk)/5)/2 + 2^(1/2)/2)^2 - 5/4)^2)^(1/2))/10 + ((cos(pi/2 + (2*pi*clk)/5)/4 + 2^(1/2)/4)*((2*pi*cos(pi/2 + (2*pi*clk)/5)*(sin(pi/2 + (2*pi*clk)/5)/2 + 2^(1/2)/2))/5 - (2*pi*sin(pi/2 + (2*pi*clk)/5)*(cos(pi/2 + (2*pi*clk)/5)/2 + 2^(1/2)/2))/5)*((cos(pi/2 + (2*pi*clk)/5)/2 + 2^(1/2)/2)^2 + (sin(pi/2 + (2*pi*clk)/5)/2 + 2^(1/2)/2)^2 - 5/4))/(1 - ((cos(pi/2 + (2*pi*clk)/5)/2 + 2^(1/2)/2)^2 + (sin(pi/2 + (2*pi*clk)/5)/2 + 2^(1/2)/2)^2 - 5/4)^2)^(1/2)))/((cos(pi/2 + (2*pi*clk)/5)/2 + 2^(1/2)/2)^2 + (sin(pi/2 + (2*pi*clk)/5)/2 + 2^(1/2)/2)^2)^2 - (2*((cos(pi/2 + (2*pi*clk)/5)/4 + 2^(1/2)/4)*(1 - ((cos(pi/2 + (2*pi*clk)/5)/2 + 2^(1/2)/2)^2 + (sin(pi/2 + (2*pi*clk)/5)/2 + 2^(1/2)/2)^2 - 5/4)^2)^(1/2) - (sin(pi/2 + (2*pi*clk)/5)/2 + 2^(1/2)/2)*((cos(pi/2 + (2*pi*clk)/5)/2 + 2^(1/2)/2)^2/2 + (sin(pi/2 + (2*pi*clk)/5)/2 + 2^(1/2)/2)^2/2 + 3/8))*((2*pi*cos(pi/2 + (2*pi*clk)/5)*(sin(pi/2 + (2*pi*clk)/5)/2 + 2^(1/2)/2))/5 - (2*pi*sin(pi/2 + (2*pi*clk)/5)*(cos(pi/2 + (2*pi*clk)/5)/2 + 2^(1/2)/2))/5)^2)/((cos(pi/2 + (2*pi*clk)/5)/2 + 2^(1/2)/2)^2 + (sin(pi/2 + (2*pi*clk)/5)/2 + 2^(1/2)/2)^2)^3 + (((cos(pi/2 + (2*pi*clk)/5)/4 + 2^(1/2)/4)*(1 - ((cos(pi/2 + (2*pi*clk)/5)/2 + 2^(1/2)/2)^2 + (sin(pi/2 + (2*pi*clk)/5)/2 + 2^(1/2)/2)^2 - 5/4)^2)^(1/2) - (sin(pi/2 + (2*pi*clk)/5)/2 + 2^(1/2)/2)*((cos(pi/2 + (2*pi*clk)/5)/2 + 2^(1/2)/2)^2/2 + (sin(pi/2 + (2*pi*clk)/5)/2 + 2^(1/2)/2)^2/2 + 3/8))*((2*pi^2*sin(pi/2 + (2*pi*clk)/5)^2)/25 + (2*pi^2*cos(pi/2 + (2*pi*clk)/5)^2)/25 - (4*pi^2*cos(pi/2 + (2*pi*clk)/5)*(cos(pi/2 + (2*pi*clk)/5)/2 + 2^(1/2)/2))/25 - (4*pi^2*sin(pi/2 + (2*pi*clk)/5)*(sin(pi/2 + (2*pi*clk)/5)/2 + 2^(1/2)/2))/25))/((cos(pi/2 + (2*pi*clk)/5)/2 + 2^(1/2)/2)^2 + (sin(pi/2 + (2*pi*clk)/5)/2 + 2^(1/2)/2)^2)^2)/(1 - ((cos(pi/2 + (2*pi*clk)/5)/4 + 2^(1/2)/4)*(1 - ((cos(pi/2 + (2*pi*clk)/5)/2 + 2^(1/2)/2)^2 + (sin(pi/2 + (2*pi*clk)/5)/2 + 2^(1/2)/2)^2 - 5/4)^2)^(1/2) - (sin(pi/2 + (2*pi*clk)/5)/2 + 2^(1/2)/2)*((cos(pi/2 + (2*pi*clk)/5)/2 + 2^(1/2)/2)^2/2 + (sin(pi/2 + (2*pi*clk)/5)/2 + 2^(1/2)/2)^2/2 + 3/8))^2/((cos(pi/2 + (2*clk*pi)/5)/2 + 2^(1/2)/2)^2 + (sin(pi/2 + (2*clk*pi)/5)/2 + 2^(1/2)/2)^2)^2)^(1/2) - ((((sin(pi/2 + (2*pi*clk)/5)/2 + 2^(1/2)/2)*((pi*cos(pi/2 + (2*pi*clk)/5)*(sin(pi/2 + (2*pi*clk)/5)/2 + 2^(1/2)/2))/5 - (pi*sin(pi/2 + (2*pi*clk)/5)*(cos(pi/2 + (2*pi*clk)/5)/2 + 2^(1/2)/2))/5) + (pi*cos(pi/2 + (2*pi*clk)/5)*((cos(pi/2 + (2*pi*clk)/5)/2 + 2^(1/2)/2)^2/2 + (sin(pi/2 + (2*pi*clk)/5)/2 + 2^(1/2)/2)^2/2 + 3/8))/5 + (pi*sin(pi/2 + (2*pi*clk)/5)*(1 - ((cos(pi/2 + (2*pi*clk)/5)/2 + 2^(1/2)/2)^2 + (sin(pi/2 + (2*pi*clk)/5)/2 + 2^(1/2)/2)^2 - 5/4)^2)^(1/2))/10 + ((cos(pi/2 + (2*pi*clk)/5)/4 + 2^(1/2)/4)*((2*pi*cos(pi/2 + (2*pi*clk)/5)*(sin(pi/2 + (2*pi*clk)/5)/2 + 2^(1/2)/2))/5 - (2*pi*sin(pi/2 + (2*pi*clk)/5)*(cos(pi/2 + (2*pi*clk)/5)/2 + 2^(1/2)/2))/5)*((cos(pi/2 + (2*pi*clk)/5)/2 + 2^(1/2)/2)^2 + (sin(pi/2 + (2*pi*clk)/5)/2 + 2^(1/2)/2)^2 - 5/4))/(1 - ((cos(pi/2 + (2*pi*clk)/5)/2 + 2^(1/2)/2)^2 + (sin(pi/2 + (2*pi*clk)/5)/2 + 2^(1/2)/2)^2 - 5/4)^2)^(1/2))/((cos(pi/2 + (2*pi*clk)/5)/2 + 2^(1/2)/2)^2 + (sin(pi/2 + (2*pi*clk)/5)/2 + 2^(1/2)/2)^2) + (((cos(pi/2 + (2*pi*clk)/5)/4 + 2^(1/2)/4)*(1 - ((cos(pi/2 + (2*pi*clk)/5)/2 + 2^(1/2)/2)^2 + (sin(pi/2 + (2*pi*clk)/5)/2 + 2^(1/2)/2)^2 - 5/4)^2)^(1/2) - (sin(pi/2 + (2*pi*clk)/5)/2 + 2^(1/2)/2)*((cos(pi/2 + (2*pi*clk)/5)/2 + 2^(1/2)/2)^2/2 + (sin(pi/2 + (2*pi*clk)/5)/2 + 2^(1/2)/2)^2/2 + 3/8))*((2*pi*cos(pi/2 + (2*pi*clk)/5)*(sin(pi/2 + (2*pi*clk)/5)/2 + 2^(1/2)/2))/5 - (2*pi*sin(pi/2 + (2*pi*clk)/5)*(cos(pi/2 + (2*pi*clk)/5)/2 + 2^(1/2)/2))/5))/((cos(pi/2 + (2*pi*clk)/5)/2 + 2^(1/2)/2)^2 + (sin(pi/2 + (2*pi*clk)/5)/2 + 2^(1/2)/2)^2)^2)*((2*((cos(pi/2 + (2*pi*clk)/5)/4 + 2^(1/2)/4)*(1 - ((cos(pi/2 + (2*pi*clk)/5)/2 + 2^(1/2)/2)^2 + (sin(pi/2 + (2*pi*clk)/5)/2 + 2^(1/2)/2)^2 - 5/4)^2)^(1/2) - (sin(pi/2 + (2*pi*clk)/5)/2 + 2^(1/2)/2)*((cos(pi/2 + (2*pi*clk)/5)/2 + 2^(1/2)/2)^2/2 + (sin(pi/2 + (2*pi*clk)/5)/2 + 2^(1/2)/2)^2/2 + 3/8))^2*((2*pi*cos(pi/2 + (2*pi*clk)/5)*(sin(pi/2 + (2*pi*clk)/5)/2 + 2^(1/2)/2))/5 - (2*pi*sin(pi/2 + (2*pi*clk)/5)*(cos(pi/2 + (2*pi*clk)/5)/2 + 2^(1/2)/2))/5))/((cos(pi/2 + (2*pi*clk)/5)/2 + 2^(1/2)/2)^2 + (sin(pi/2 + (2*pi*clk)/5)/2 + 2^(1/2)/2)^2)^3 + (2*((cos(pi/2 + (2*pi*clk)/5)/4 + 2^(1/2)/4)*(1 - ((cos(pi/2 + (2*pi*clk)/5)/2 + 2^(1/2)/2)^2 + (sin(pi/2 + (2*pi*clk)/5)/2 + 2^(1/2)/2)^2 - 5/4)^2)^(1/2) - (sin(pi/2 + (2*pi*clk)/5)/2 + 2^(1/2)/2)*((cos(pi/2 + (2*pi*clk)/5)/2 + 2^(1/2)/2)^2/2 + (sin(pi/2 + (2*pi*clk)/5)/2 + 2^(1/2)/2)^2/2 + 3/8))*((sin(pi/2 + (2*pi*clk)/5)/2 + 2^(1/2)/2)*((pi*cos(pi/2 + (2*pi*clk)/5)*(sin(pi/2 + (2*pi*clk)/5)/2 + 2^(1/2)/2))/5 - (pi*sin(pi/2 + (2*pi*clk)/5)*(cos(pi/2 + (2*pi*clk)/5)/2 + 2^(1/2)/2))/5) + (pi*cos(pi/2 + (2*pi*clk)/5)*((cos(pi/2 + (2*pi*clk)/5)/2 + 2^(1/2)/2)^2/2 + (sin(pi/2 + (2*pi*clk)/5)/2 + 2^(1/2)/2)^2/2 + 3/8))/5 + (pi*sin(pi/2 + (2*pi*clk)/5)*(1 - ((cos(pi/2 + (2*pi*clk)/5)/2 + 2^(1/2)/2)^2 + (sin(pi/2 + (2*pi*clk)/5)/2 + 2^(1/2)/2)^2 - 5/4)^2)^(1/2))/10 + ((cos(pi/2 + (2*pi*clk)/5)/4 + 2^(1/2)/4)*((2*pi*cos(pi/2 + (2*pi*clk)/5)*(sin(pi/2 + (2*pi*clk)/5)/2 + 2^(1/2)/2))/5 - (2*pi*sin(pi/2 + (2*pi*clk)/5)*(cos(pi/2 + (2*pi*clk)/5)/2 + 2^(1/2)/2))/5)*((cos(pi/2 + (2*pi*clk)/5)/2 + 2^(1/2)/2)^2 + (sin(pi/2 + (2*pi*clk)/5)/2 + 2^(1/2)/2)^2 - 5/4))/(1 - ((cos(pi/2 + (2*pi*clk)/5)/2 + 2^(1/2)/2)^2 + (sin(pi/2 + (2*pi*clk)/5)/2 + 2^(1/2)/2)^2 - 5/4)^2)^(1/2)))/((cos(pi/2 + (2*pi*clk)/5)/2 + 2^(1/2)/2)^2 + (sin(pi/2 + (2*pi*clk)/5)/2 + 2^(1/2)/2)^2)^2))/(2*(1 - ((cos(pi/2 + (2*pi*clk)/5)/4 + 2^(1/2)/4)*(1 - ((cos(pi/2 + (2*pi*clk)/5)/2 + 2^(1/2)/2)^2 + (sin(pi/2 + (2*pi*clk)/5)/2 + 2^(1/2)/2)^2 - 5/4)^2)^(1/2) - (sin(pi/2 + (2*pi*clk)/5)/2 + 2^(1/2)/2)*((cos(pi/2 + (2*pi*clk)/5)/2 + 2^(1/2)/2)^2/2 + (sin(pi/2 + (2*pi*clk)/5)/2 + 2^(1/2)/2)^2/2 + 3/8))^2/((cos(pi/2 + (2*clk*pi)/5)/2 + 2^(1/2)/2)^2 + (sin(pi/2 + (2*clk*pi)/5)/2 + 2^(1/2)/2)^2)^2)^(3/2));
    
       else
            qd1 = pi- qd1;
            qd1_dot = -(((sin(pi/2 + (2*pi*clk)/5)/2 + 2^(1/2)/2)*((pi*cos(pi/2 + (2*pi*clk)/5)*(sin(pi/2 + (2*pi*clk)/5)/2 + 2^(1/2)/2))/5 - (pi*sin(pi/2 + (2*pi*clk)/5)*(cos(pi/2 + (2*pi*clk)/5)/2 + 2^(1/2)/2))/5) + (pi*cos(pi/2 + (2*pi*clk)/5)*((cos(pi/2 + (2*pi*clk)/5)/2 + 2^(1/2)/2)^2/2 + (sin(pi/2 + (2*pi*clk)/5)/2 + 2^(1/2)/2)^2/2 + 3/8))/5 + (pi*sin(pi/2 + (2*pi*clk)/5)*(1 - ((cos(pi/2 + (2*pi*clk)/5)/2 + 2^(1/2)/2)^2 + (sin(pi/2 + (2*pi*clk)/5)/2 + 2^(1/2)/2)^2 - 5/4)^2)^(1/2))/10 + ((cos(pi/2 + (2*pi*clk)/5)/4 + 2^(1/2)/4)*((2*pi*cos(pi/2 + (2*pi*clk)/5)*(sin(pi/2 + (2*pi*clk)/5)/2 + 2^(1/2)/2))/5 - (2*pi*sin(pi/2 + (2*pi*clk)/5)*(cos(pi/2 + (2*pi*clk)/5)/2 + 2^(1/2)/2))/5)*((cos(pi/2 + (2*pi*clk)/5)/2 + 2^(1/2)/2)^2 + (sin(pi/2 + (2*pi*clk)/5)/2 + 2^(1/2)/2)^2 - 5/4))/(1 - ((cos(pi/2 + (2*pi*clk)/5)/2 + 2^(1/2)/2)^2 + (sin(pi/2 + (2*pi*clk)/5)/2 + 2^(1/2)/2)^2 - 5/4)^2)^(1/2))/((cos(pi/2 + (2*pi*clk)/5)/2 + 2^(1/2)/2)^2 + (sin(pi/2 + (2*pi*clk)/5)/2 + 2^(1/2)/2)^2) + (((cos(pi/2 + (2*pi*clk)/5)/4 + 2^(1/2)/4)*(1 - ((cos(pi/2 + (2*pi*clk)/5)/2 + 2^(1/2)/2)^2 + (sin(pi/2 + (2*pi*clk)/5)/2 + 2^(1/2)/2)^2 - 5/4)^2)^(1/2) - (sin(pi/2 + (2*pi*clk)/5)/2 + 2^(1/2)/2)*((cos(pi/2 + (2*pi*clk)/5)/2 + 2^(1/2)/2)^2/2 + (sin(pi/2 + (2*pi*clk)/5)/2 + 2^(1/2)/2)^2/2 + 3/8))*((2*pi*cos(pi/2 + (2*pi*clk)/5)*(sin(pi/2 + (2*pi*clk)/5)/2 + 2^(1/2)/2))/5 - (2*pi*sin(pi/2 + (2*pi*clk)/5)*(cos(pi/2 + (2*pi*clk)/5)/2 + 2^(1/2)/2))/5))/((cos(pi/2 + (2*pi*clk)/5)/2 + 2^(1/2)/2)^2 + (sin(pi/2 + (2*pi*clk)/5)/2 + 2^(1/2)/2)^2)^2)/(1 - ((cos(pi/2 + (2*pi*clk)/5)/4 + 2^(1/2)/4)*(1 - ((cos(pi/2 + (2*pi*clk)/5)/2 + 2^(1/2)/2)^2 + (sin(pi/2 + (2*pi*clk)/5)/2 + 2^(1/2)/2)^2 - 5/4)^2)^(1/2) - (sin(pi/2 + (2*pi*clk)/5)/2 + 2^(1/2)/2)*((cos(pi/2 + (2*pi*clk)/5)/2 + 2^(1/2)/2)^2/2 + (sin(pi/2 + (2*pi*clk)/5)/2 + 2^(1/2)/2)^2/2 + 3/8))^2/((cos(pi/2 + (2*clk*pi)/5)/2 + 2^(1/2)/2)^2 + (sin(pi/2 + (2*clk*pi)/5)/2 + 2^(1/2)/2)^2)^2)^(1/2);
            qd1_dotdot = ((((sin(pi/2 + (2*pi*clk)/5)/2 + 2^(1/2)/2)*((pi*cos(pi/2 + (2*pi*clk)/5)*(sin(pi/2 + (2*pi*clk)/5)/2 + 2^(1/2)/2))/5 - (pi*sin(pi/2 + (2*pi*clk)/5)*(cos(pi/2 + (2*pi*clk)/5)/2 + 2^(1/2)/2))/5) + (pi*cos(pi/2 + (2*pi*clk)/5)*((cos(pi/2 + (2*pi*clk)/5)/2 + 2^(1/2)/2)^2/2 + (sin(pi/2 + (2*pi*clk)/5)/2 + 2^(1/2)/2)^2/2 + 3/8))/5 + (pi*sin(pi/2 + (2*pi*clk)/5)*(1 - ((cos(pi/2 + (2*pi*clk)/5)/2 + 2^(1/2)/2)^2 + (sin(pi/2 + (2*pi*clk)/5)/2 + 2^(1/2)/2)^2 - 5/4)^2)^(1/2))/10 + ((cos(pi/2 + (2*pi*clk)/5)/4 + 2^(1/2)/4)*((2*pi*cos(pi/2 + (2*pi*clk)/5)*(sin(pi/2 + (2*pi*clk)/5)/2 + 2^(1/2)/2))/5 - (2*pi*sin(pi/2 + (2*pi*clk)/5)*(cos(pi/2 + (2*pi*clk)/5)/2 + 2^(1/2)/2))/5)*((cos(pi/2 + (2*pi*clk)/5)/2 + 2^(1/2)/2)^2 + (sin(pi/2 + (2*pi*clk)/5)/2 + 2^(1/2)/2)^2 - 5/4))/(1 - ((cos(pi/2 + (2*pi*clk)/5)/2 + 2^(1/2)/2)^2 + (sin(pi/2 + (2*pi*clk)/5)/2 + 2^(1/2)/2)^2 - 5/4)^2)^(1/2))/((cos(pi/2 + (2*pi*clk)/5)/2 + 2^(1/2)/2)^2 + (sin(pi/2 + (2*pi*clk)/5)/2 + 2^(1/2)/2)^2) + (((cos(pi/2 + (2*pi*clk)/5)/4 + 2^(1/2)/4)*(1 - ((cos(pi/2 + (2*pi*clk)/5)/2 + 2^(1/2)/2)^2 + (sin(pi/2 + (2*pi*clk)/5)/2 + 2^(1/2)/2)^2 - 5/4)^2)^(1/2) - (sin(pi/2 + (2*pi*clk)/5)/2 + 2^(1/2)/2)*((cos(pi/2 + (2*pi*clk)/5)/2 + 2^(1/2)/2)^2/2 + (sin(pi/2 + (2*pi*clk)/5)/2 + 2^(1/2)/2)^2/2 + 3/8))*((2*pi*cos(pi/2 + (2*pi*clk)/5)*(sin(pi/2 + (2*pi*clk)/5)/2 + 2^(1/2)/2))/5 - (2*pi*sin(pi/2 + (2*pi*clk)/5)*(cos(pi/2 + (2*pi*clk)/5)/2 + 2^(1/2)/2))/5))/((cos(pi/2 + (2*pi*clk)/5)/2 + 2^(1/2)/2)^2 + (sin(pi/2 + (2*pi*clk)/5)/2 + 2^(1/2)/2)^2)^2)*((2*((cos(pi/2 + (2*pi*clk)/5)/4 + 2^(1/2)/4)*(1 - ((cos(pi/2 + (2*pi*clk)/5)/2 + 2^(1/2)/2)^2 + (sin(pi/2 + (2*pi*clk)/5)/2 + 2^(1/2)/2)^2 - 5/4)^2)^(1/2) - (sin(pi/2 + (2*pi*clk)/5)/2 + 2^(1/2)/2)*((cos(pi/2 + (2*pi*clk)/5)/2 + 2^(1/2)/2)^2/2 + (sin(pi/2 + (2*pi*clk)/5)/2 + 2^(1/2)/2)^2/2 + 3/8))^2*((2*pi*cos(pi/2 + (2*pi*clk)/5)*(sin(pi/2 + (2*pi*clk)/5)/2 + 2^(1/2)/2))/5 - (2*pi*sin(pi/2 + (2*pi*clk)/5)*(cos(pi/2 + (2*pi*clk)/5)/2 + 2^(1/2)/2))/5))/((cos(pi/2 + (2*pi*clk)/5)/2 + 2^(1/2)/2)^2 + (sin(pi/2 + (2*pi*clk)/5)/2 + 2^(1/2)/2)^2)^3 + (2*((cos(pi/2 + (2*pi*clk)/5)/4 + 2^(1/2)/4)*(1 - ((cos(pi/2 + (2*pi*clk)/5)/2 + 2^(1/2)/2)^2 + (sin(pi/2 + (2*pi*clk)/5)/2 + 2^(1/2)/2)^2 - 5/4)^2)^(1/2) - (sin(pi/2 + (2*pi*clk)/5)/2 + 2^(1/2)/2)*((cos(pi/2 + (2*pi*clk)/5)/2 + 2^(1/2)/2)^2/2 + (sin(pi/2 + (2*pi*clk)/5)/2 + 2^(1/2)/2)^2/2 + 3/8))*((sin(pi/2 + (2*pi*clk)/5)/2 + 2^(1/2)/2)*((pi*cos(pi/2 + (2*pi*clk)/5)*(sin(pi/2 + (2*pi*clk)/5)/2 + 2^(1/2)/2))/5 - (pi*sin(pi/2 + (2*pi*clk)/5)*(cos(pi/2 + (2*pi*clk)/5)/2 + 2^(1/2)/2))/5) + (pi*cos(pi/2 + (2*pi*clk)/5)*((cos(pi/2 + (2*pi*clk)/5)/2 + 2^(1/2)/2)^2/2 + (sin(pi/2 + (2*pi*clk)/5)/2 + 2^(1/2)/2)^2/2 + 3/8))/5 + (pi*sin(pi/2 + (2*pi*clk)/5)*(1 - ((cos(pi/2 + (2*pi*clk)/5)/2 + 2^(1/2)/2)^2 + (sin(pi/2 + (2*pi*clk)/5)/2 + 2^(1/2)/2)^2 - 5/4)^2)^(1/2))/10 + ((cos(pi/2 + (2*pi*clk)/5)/4 + 2^(1/2)/4)*((2*pi*cos(pi/2 + (2*pi*clk)/5)*(sin(pi/2 + (2*pi*clk)/5)/2 + 2^(1/2)/2))/5 - (2*pi*sin(pi/2 + (2*pi*clk)/5)*(cos(pi/2 + (2*pi*clk)/5)/2 + 2^(1/2)/2))/5)*((cos(pi/2 + (2*pi*clk)/5)/2 + 2^(1/2)/2)^2 + (sin(pi/2 + (2*pi*clk)/5)/2 + 2^(1/2)/2)^2 - 5/4))/(1 - ((cos(pi/2 + (2*pi*clk)/5)/2 + 2^(1/2)/2)^2 + (sin(pi/2 + (2*pi*clk)/5)/2 + 2^(1/2)/2)^2 - 5/4)^2)^(1/2)))/((cos(pi/2 + (2*pi*clk)/5)/2 + 2^(1/2)/2)^2 + (sin(pi/2 + (2*pi*clk)/5)/2 + 2^(1/2)/2)^2)^2))/(2*(1 - ((cos(pi/2 + (2*pi*clk)/5)/4 + 2^(1/2)/4)*(1 - ((cos(pi/2 + (2*pi*clk)/5)/2 + 2^(1/2)/2)^2 + (sin(pi/2 + (2*pi*clk)/5)/2 + 2^(1/2)/2)^2 - 5/4)^2)^(1/2) - (sin(pi/2 + (2*pi*clk)/5)/2 + 2^(1/2)/2)*((cos(pi/2 + (2*pi*clk)/5)/2 + 2^(1/2)/2)^2/2 + (sin(pi/2 + (2*pi*clk)/5)/2 + 2^(1/2)/2)^2/2 + 3/8))^2/((cos(pi/2 + (2*clk*pi)/5)/2 + 2^(1/2)/2)^2 + (sin(pi/2 + (2*clk*pi)/5)/2 + 2^(1/2)/2)^2)^2)^(3/2)) - (((sin(pi/2 + (2*pi*clk)/5)/2 + 2^(1/2)/2)*((pi^2*sin(pi/2 + (2*pi*clk)/5)^2)/25 + (pi^2*cos(pi/2 + (2*pi*clk)/5)^2)/25 - (2*pi^2*cos(pi/2 + (2*pi*clk)/5)*(cos(pi/2 + (2*pi*clk)/5)/2 + 2^(1/2)/2))/25 - (2*pi^2*sin(pi/2 + (2*pi*clk)/5)*(sin(pi/2 + (2*pi*clk)/5)/2 + 2^(1/2)/2))/25) + (2*pi*cos(pi/2 + (2*pi*clk)/5)*((pi*cos(pi/2 + (2*pi*clk)/5)*(sin(pi/2 + (2*pi*clk)/5)/2 + 2^(1/2)/2))/5 - (pi*sin(pi/2 + (2*pi*clk)/5)*(cos(pi/2 + (2*pi*clk)/5)/2 + 2^(1/2)/2))/5))/5 + (pi^2*cos(pi/2 + (2*pi*clk)/5)*(1 - ((cos(pi/2 + (2*pi*clk)/5)/2 + 2^(1/2)/2)^2 + (sin(pi/2 + (2*pi*clk)/5)/2 + 2^(1/2)/2)^2 - 5/4)^2)^(1/2))/25 + ((cos(pi/2 + (2*pi*clk)/5)/4 + 2^(1/2)/4)*((2*pi*cos(pi/2 + (2*pi*clk)/5)*(sin(pi/2 + (2*pi*clk)/5)/2 + 2^(1/2)/2))/5 - (2*pi*sin(pi/2 + (2*pi*clk)/5)*(cos(pi/2 + (2*pi*clk)/5)/2 + 2^(1/2)/2))/5)^2)/(1 - ((cos(pi/2 + (2*pi*clk)/5)/2 + 2^(1/2)/2)^2 + (sin(pi/2 + (2*pi*clk)/5)/2 + 2^(1/2)/2)^2 - 5/4)^2)^(1/2) - (2*pi^2*sin(pi/2 + (2*pi*clk)/5)*((cos(pi/2 + (2*pi*clk)/5)/2 + 2^(1/2)/2)^2/2 + (sin(pi/2 + (2*pi*clk)/5)/2 + 2^(1/2)/2)^2/2 + 3/8))/25 + ((cos(pi/2 + (2*pi*clk)/5)/4 + 2^(1/2)/4)*((cos(pi/2 + (2*pi*clk)/5)/2 + 2^(1/2)/2)^2 + (sin(pi/2 + (2*pi*clk)/5)/2 + 2^(1/2)/2)^2 - 5/4)*((2*pi^2*sin(pi/2 + (2*pi*clk)/5)^2)/25 + (2*pi^2*cos(pi/2 + (2*pi*clk)/5)^2)/25 - (4*pi^2*cos(pi/2 + (2*pi*clk)/5)*(cos(pi/2 + (2*pi*clk)/5)/2 + 2^(1/2)/2))/25 - (4*pi^2*sin(pi/2 + (2*pi*clk)/5)*(sin(pi/2 + (2*pi*clk)/5)/2 + 2^(1/2)/2))/25))/(1 - ((cos(pi/2 + (2*pi*clk)/5)/2 + 2^(1/2)/2)^2 + (sin(pi/2 + (2*pi*clk)/5)/2 + 2^(1/2)/2)^2 - 5/4)^2)^(1/2) + ((cos(pi/2 + (2*pi*clk)/5)/4 + 2^(1/2)/4)*((2*pi*cos(pi/2 + (2*pi*clk)/5)*(sin(pi/2 + (2*pi*clk)/5)/2 + 2^(1/2)/2))/5 - (2*pi*sin(pi/2 + (2*pi*clk)/5)*(cos(pi/2 + (2*pi*clk)/5)/2 + 2^(1/2)/2))/5)^2*((cos(pi/2 + (2*pi*clk)/5)/2 + 2^(1/2)/2)^2 + (sin(pi/2 + (2*pi*clk)/5)/2 + 2^(1/2)/2)^2 - 5/4)^2)/(1 - ((cos(pi/2 + (2*pi*clk)/5)/2 + 2^(1/2)/2)^2 + (sin(pi/2 + (2*pi*clk)/5)/2 + 2^(1/2)/2)^2 - 5/4)^2)^(3/2) - (pi*sin(pi/2 + (2*pi*clk)/5)*((2*pi*cos(pi/2 + (2*pi*clk)/5)*(sin(pi/2 + (2*pi*clk)/5)/2 + 2^(1/2)/2))/5 - (2*pi*sin(pi/2 + (2*pi*clk)/5)*(cos(pi/2 + (2*pi*clk)/5)/2 + 2^(1/2)/2))/5)*((cos(pi/2 + (2*pi*clk)/5)/2 + 2^(1/2)/2)^2 + (sin(pi/2 + (2*pi*clk)/5)/2 + 2^(1/2)/2)^2 - 5/4))/(5*(1 - ((cos(pi/2 + (2*pi*clk)/5)/2 + 2^(1/2)/2)^2 + (sin(pi/2 + (2*pi*clk)/5)/2 + 2^(1/2)/2)^2 - 5/4)^2)^(1/2)))/((cos(pi/2 + (2*pi*clk)/5)/2 + 2^(1/2)/2)^2 + (sin(pi/2 + (2*pi*clk)/5)/2 + 2^(1/2)/2)^2) - (2*((2*pi*cos(pi/2 + (2*pi*clk)/5)*(sin(pi/2 + (2*pi*clk)/5)/2 + 2^(1/2)/2))/5 - (2*pi*sin(pi/2 + (2*pi*clk)/5)*(cos(pi/2 + (2*pi*clk)/5)/2 + 2^(1/2)/2))/5)*((sin(pi/2 + (2*pi*clk)/5)/2 + 2^(1/2)/2)*((pi*cos(pi/2 + (2*pi*clk)/5)*(sin(pi/2 + (2*pi*clk)/5)/2 + 2^(1/2)/2))/5 - (pi*sin(pi/2 + (2*pi*clk)/5)*(cos(pi/2 + (2*pi*clk)/5)/2 + 2^(1/2)/2))/5) + (pi*cos(pi/2 + (2*pi*clk)/5)*((cos(pi/2 + (2*pi*clk)/5)/2 + 2^(1/2)/2)^2/2 + (sin(pi/2 + (2*pi*clk)/5)/2 + 2^(1/2)/2)^2/2 + 3/8))/5 + (pi*sin(pi/2 + (2*pi*clk)/5)*(1 - ((cos(pi/2 + (2*pi*clk)/5)/2 + 2^(1/2)/2)^2 + (sin(pi/2 + (2*pi*clk)/5)/2 + 2^(1/2)/2)^2 - 5/4)^2)^(1/2))/10 + ((cos(pi/2 + (2*pi*clk)/5)/4 + 2^(1/2)/4)*((2*pi*cos(pi/2 + (2*pi*clk)/5)*(sin(pi/2 + (2*pi*clk)/5)/2 + 2^(1/2)/2))/5 - (2*pi*sin(pi/2 + (2*pi*clk)/5)*(cos(pi/2 + (2*pi*clk)/5)/2 + 2^(1/2)/2))/5)*((cos(pi/2 + (2*pi*clk)/5)/2 + 2^(1/2)/2)^2 + (sin(pi/2 + (2*pi*clk)/5)/2 + 2^(1/2)/2)^2 - 5/4))/(1 - ((cos(pi/2 + (2*pi*clk)/5)/2 + 2^(1/2)/2)^2 + (sin(pi/2 + (2*pi*clk)/5)/2 + 2^(1/2)/2)^2 - 5/4)^2)^(1/2)))/((cos(pi/2 + (2*pi*clk)/5)/2 + 2^(1/2)/2)^2 + (sin(pi/2 + (2*pi*clk)/5)/2 + 2^(1/2)/2)^2)^2 - (2*((cos(pi/2 + (2*pi*clk)/5)/4 + 2^(1/2)/4)*(1 - ((cos(pi/2 + (2*pi*clk)/5)/2 + 2^(1/2)/2)^2 + (sin(pi/2 + (2*pi*clk)/5)/2 + 2^(1/2)/2)^2 - 5/4)^2)^(1/2) - (sin(pi/2 + (2*pi*clk)/5)/2 + 2^(1/2)/2)*((cos(pi/2 + (2*pi*clk)/5)/2 + 2^(1/2)/2)^2/2 + (sin(pi/2 + (2*pi*clk)/5)/2 + 2^(1/2)/2)^2/2 + 3/8))*((2*pi*cos(pi/2 + (2*pi*clk)/5)*(sin(pi/2 + (2*pi*clk)/5)/2 + 2^(1/2)/2))/5 - (2*pi*sin(pi/2 + (2*pi*clk)/5)*(cos(pi/2 + (2*pi*clk)/5)/2 + 2^(1/2)/2))/5)^2)/((cos(pi/2 + (2*pi*clk)/5)/2 + 2^(1/2)/2)^2 + (sin(pi/2 + (2*pi*clk)/5)/2 + 2^(1/2)/2)^2)^3 + (((cos(pi/2 + (2*pi*clk)/5)/4 + 2^(1/2)/4)*(1 - ((cos(pi/2 + (2*pi*clk)/5)/2 + 2^(1/2)/2)^2 + (sin(pi/2 + (2*pi*clk)/5)/2 + 2^(1/2)/2)^2 - 5/4)^2)^(1/2) - (sin(pi/2 + (2*pi*clk)/5)/2 + 2^(1/2)/2)*((cos(pi/2 + (2*pi*clk)/5)/2 + 2^(1/2)/2)^2/2 + (sin(pi/2 + (2*pi*clk)/5)/2 + 2^(1/2)/2)^2/2 + 3/8))*((2*pi^2*sin(pi/2 + (2*pi*clk)/5)^2)/25 + (2*pi^2*cos(pi/2 + (2*pi*clk)/5)^2)/25 - (4*pi^2*cos(pi/2 + (2*pi*clk)/5)*(cos(pi/2 + (2*pi*clk)/5)/2 + 2^(1/2)/2))/25 - (4*pi^2*sin(pi/2 + (2*pi*clk)/5)*(sin(pi/2 + (2*pi*clk)/5)/2 + 2^(1/2)/2))/25))/((cos(pi/2 + (2*pi*clk)/5)/2 + 2^(1/2)/2)^2 + (sin(pi/2 + (2*pi*clk)/5)/2 + 2^(1/2)/2)^2)^2)/(1 - ((cos(pi/2 + (2*pi*clk)/5)/4 + 2^(1/2)/4)*(1 - ((cos(pi/2 + (2*pi*clk)/5)/2 + 2^(1/2)/2)^2 + (sin(pi/2 + (2*pi*clk)/5)/2 + 2^(1/2)/2)^2 - 5/4)^2)^(1/2) - (sin(pi/2 + (2*pi*clk)/5)/2 + 2^(1/2)/2)*((cos(pi/2 + (2*pi*clk)/5)/2 + 2^(1/2)/2)^2/2 + (sin(pi/2 + (2*pi*clk)/5)/2 + 2^(1/2)/2)^2/2 + 3/8))^2/((cos(pi/2 + (2*clk*pi)/5)/2 + 2^(1/2)/2)^2 + (sin(pi/2 + (2*clk*pi)/5)/2 + 2^(1/2)/2)^2)^2)^(1/2);
     
       end
end

== matlab function Computed Torque Controller/Neural Network /RBF for q1 ==
  data: qa1 input double; qa1_dot input double; qda1 input double; qda1_dot input double; Tnn1 output double
function Tnn1    = NeuralNetwork(qa1,qa1_dot,qda1,qda1_dot)
N=121;
M = sqrt(N);
persistent  X C var centerx centery CENTER_X CENTER_Y


%% Initialize the weighted matrices
if isempty(C)
    C = 0.1*ones(N,1);              % Output weight
    var = 0.141*ones(N,1);        % variance (sigma)
    centerx = -0.1:0.02:0.1;        % centers
    centery = -3:0.6:3;
    X = ones(2,1);                     % Input
   [CENTER_X,CENTER_Y] = meshgrid(centerx,centery);
end

%% Input of neural network

x1 = qa1 - qda1;                       % error
x2 = qa1_dot - qda1_dot;           % error_dot

X(1) = x1;
X(2) = x2;

  


%% Replaced function
% lamda1 = 0.005;
% s1 = (qa1 - qda1) + lamda1*(qa1_dot - qda1_dot);
lamda1 =  0.5;
lamda2 = 15;
% lamda1 =  1;
% lamda2 = 15;
s1 = (qa1 - qda1)*lamda2 + lamda1*(qa1_dot - qda1_dot);
S = s1;


%% HIDDEN LAYER (The basis function is chosen as Gaussian function)

R_temp = zeros(M,M);

for i = 1:10
    for j = 1:10
        R_temp(i,j) = (X(1)-CENTER_X(i,j))^2 + (X(2)-CENTER_Y(i,j))^2;
         R_temp(i,j) =  (R_temp(i,j)/(var(i*M-M+j)^2))/2;
          R_temp(i,j) = exp(-R_temp(i,j));
%R_temp(i,j) = exp(-(norm(X(1),CENTER_X(i,j))/var(i*5+j-5))^2/2)* exp(-(norm(X(2),CENTER_Y(i,j))/var(i*5+j-5))^2/2);
    end
end

% Create row(column) vector
k = 1;
Rx = zeros(1,N);
for i=1:M
    for j=1:M
    Rx(k) = R_temp(i,j);
    k= k+1;
    end
end

%% OUTPUT LAYER
T_net = zeros(1,1);
    for j=1:N
        T_net = T_net + C(j)*Rx(j);
    end



%% UPDATE WEIGHTS 
    % Learning rate
    m = 0.1; % weight learning rate
    n = 0.05; % center learning rate
    sg = 0.1; % sigma learing rate
  
% Update for ouput weights
for j = 1:N
    
       C(j) = C(j) - m*abs(S)*C(j) - m*S*Rx(j);
end

%Update for centers
for j = 1:N
    CENTER_X(j)  =  CENTER_X(j) - n*(S)*CENTER_X(j);
    CENTER_Y(j)  =  CENTER_Y(j) - n*(S)*CENTER_Y(j);
end

%Update for variance
for j = 1:N
   var(j) = var(j) - sg*S*var(j);
end

Tnn1 = T_net;
end
